simulink model "usrp_save_raw_data"  (R2017a)
settings: Solver=VariableStepAuto  StartTime=0.0  StopTime=inf  RelTol=1e-3
libraries: commsdrhw_v2 x1
settings Model: Creator=Sky  LastModifiedBy=Sky

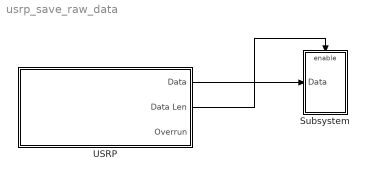
== system usrp_save_raw_data ==
  Subsystem : Subsystem
  USRP : Subsystem  mask{decimInterp=500, frameLength=100e6/500/400*3*5}
      mask prompts: decimInterp "Decimation Factor"
      mask TypeOptions decimInterp: SDRu Receiver/decimInterp
      mask TypeOptions frameLength: SDRu Receiver/frameLength
  wires:
  USRP/2(Data Len) -> Subsystem/Enable
  USRP/1(Data) -> Subsystem/1(Data)

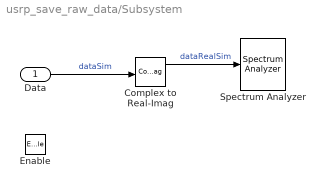
== system usrp_save_raw_data/Subsystem ==
  Data : Inport
  Enable : EnablePort
  Complex to Real-Imag : ComplexToRealImag
  Spectrum Analyzer : SpectrumAnalyzer
  wires:
  Complex to Real-Imag/1 -> Spectrum Analyzer/1  "dataRealSim"
  Data/1 -> Complex to Real-Imag/1  "dataSim"

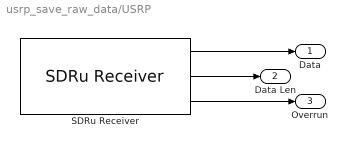
== system usrp_save_raw_data/USRP ==
  SDRu Receiver : commsdrhw_v2/SDRu Receiver  SourceLibraryInfo="This block requires <a href=\"http://www.mathworks.com/hardware-support/usrp.html\">Communications System Toolbox Support Package for USRP Radio</a>"  rxtx=rx  platform=N200/N210/USRP2  USRP2_IP='192.168.10.6'  USRP_IP_X300='192.168.10.2'  USRP_IP_X310='192.168.10.2'  USRP_serialNumB200=''  USRP_serialNumB210=''  ChannelMapping=1  centerFrequency=0  centerFrequencySrc=Dialog  loOffset=0  loOffsetSrc=Dialog  PPSSource=Internal  clockSource=Internal  masterClkRateB200=32e6  masterClkRateB210=32e6  masterClkRateX300=200e6  masterClkRateX310=200e6  masterClkRateParam=100e6  gain=0  gainSrc=Dialog  decimInterpSrc=Dialog  decimInterp=decimInterp  TransportDataType=int16  USRP2_IP_NUM=[49 57 50 46 49 54 56 46 49 48 46 54]  frameLength=frameLength  outputDatatype=single  overrunUnderrunPort=on  sampleTime=decimInterp/100e6  HOST_DATA_PORT=0  HOST_CONTROL_PORT=0  USRP2_DATA_PORT=0  USRP2_CONTROL_PORT=0  bufferMode=Continuous streaming  EnableBurstMode=off  NumFramesInBurst=10000  USRP_ID='192.168.10.6'
      settings: SourceProductName=Communications System Toolbox Support Package for USRP(R) Radio  SourceProductBaseCode=USRP
  Data : Outport
  Data Len : Outport  Port=2
  Overrun : Outport  Port=3
  wires:
  SDRu Receiver/2 -> Data Len/1
  SDRu Receiver/3 -> Overrun/1
  SDRu Receiver/1 -> Data/1
